simulink model "ATRIAS_vnmc"  (R2015a)
settings: Solver=ode45  StartTime=0.0  StopTime=60  FixedStep=1e-3  MinStep=1e-6  RelTol=1e-3  AbsTol=1e-4
values from neighbouring files (symbols this model uses):
  initial_boom_yaw = initial_boom_yaw + delta_yaw0    [run_model.m]
  max_floor_diff = cost_fun_opts.max_floor_diff    [opt_cmaes.m]    (also in run_model.m; set_all_params_simple.m = 0)
  noise_on_off = cost_fun_opts.noise_on_off    [opt_cmaes.m]    (also in run_model.m; set_all_params_simple.m = 0)
  noise_seed = cost_fun_opts.noise_seed    [opt_cmaes.m]    (also in run_model.m; set_all_params_simple.m = 1)
  noise_variance = cost_fun_opts.noise_variance    [opt_cmaes.m]    (also in run_model.m; set_all_params_simple.m = 0.000174532925199)
  SEA_swing_ctrl_on_off = cost_fun_opts.SEA_swing_ctrl_on_off    [opt_cmaes.m]    (also in run_model.m; set_all_params_simple.m = 0)
  sim_t = simout.twalk    [run_model.m]
  steady_dist = cost_fun_opts.steady_dist    [opt_cmaes.m]    (also in run_model.m; set_all_params_simple.m = 10)
  ts_anim = 0.0333    [run_model.m]
undefined symbols (not defined in the file or in its folder): A1_notch_f1, A2_notch_f1, A_lpf_dtau, A_lpf_velocity, B1_lpf_dtau, B1_lpf_velocity, B1_notch_f1, B2_lpf_dtau, B2_lpf_velocity, B2_notch_f1, b_hmotor, b_leg_spring, b_rotor, base_color_d, boom_color_d, boom_mount_to_center_diagonal, breakaway_friction, c, c_jointstop, com_height_offset, contactThr, coulomb_friction, CtrlPar_theta0, D12_S, D12_T, d_com, ddx_max, ddy_max, delta_phi_max, delta_phi_max_buffer, delta_phi_max_dropoff, delta_phi_min, des_forward_velocity, DS_width, dtau_des_max, dtheta0_vmc, dx0_vmc, dy_max, eref, fblink_color_d, fcut_acceleration, floor_color_d, floor_tile_width, floor_zero_height, FmaxBFSH, FmaxGLU, FmaxHAM, FmaxHFL, FmaxRF, FmaxVAS, FPCtrlPar, friction_linear_zone, g, gain_nodes_sea_torque, gamma_stance_thr, gamma_swing_thr, hip_height, HIP_MTR_MAX_CONT_TORQUE, HIP_MTR_MAX_TORQUE, hshaft_color_d ... (+236)
libraries: sm_lib x280, nesl_utility x174, simulink x114, simulink_extras x58, fl_lib x16, mblibv1 x2, dspswit3 x2
(part 23 of 23)

== matlab function ATRIAS_vnmc/control/Virtual Model Control/Swing Leg Behavior1/Avoid Hitting Mechanical Limits ==
  settings: updateMethod=DISCRETE  sampleTime=sample_time
  data: back_cmd output double; front_cmd output double; dback_cmd output double; dfront_cmd output double; ddback_cmd output double; ddfront_cmd output double; back_desired input; dback_desired input; ddback_desired input; front_desired input; dfront_desired input; ddfront_desired input; min_front_bar_angle parameter; max_front_bar_angle parameter; min_back_bar_angle parameter; max_back_bar_angle parameter
%% Avoid joint limits by ensuring we don't command velocities/accelerations that would push us into them when we are close to them.
function [back_cmd, front_cmd, dback_cmd, dfront_cmd, ddback_cmd, ddfront_cmd] ...
    = AvoidFourbarLimits(back_desired,dback_desired, ddback_desired, ...
          front_desired, dfront_desired, ddfront_desired, ...
          min_front_bar_angle, max_front_bar_angle, min_back_bar_angle, max_back_bar_angle)
    [back_cmd, front_cmd, dback_cmd, dfront_cmd, ddback_cmd, ddfront_cmd] = AvoidFourbarLimits(back_desired,dback_desired, ddback_desired, front_desired, dfront_desired, ddfront_desired, min_front_bar_angle, max_front_bar_angle, min_back_bar_angle, max_back_bar_angle);
end

== matlab function ATRIAS_vnmc/control/Virtual Model Control/Swing Leg Behavior1/Leg Angle Trajectory ==
  settings: updateMethod=DISCRETE  sampleTime=sample_time
  data: t input double; gamma_initial input double; gamma_final input double; t_trajectory input double; gamma output double; dgamma output double; ddgamma output double; max_gamma_velocity input; max_gamma_acceleration input
function [gamma, dgamma, ddgamma] = ...
    LegAngleTrajectory(t, gamma_initial, gamma_final, t_trajectory,...
                        max_gamma_velocity, max_gamma_acceleration)
                    
    t = max(0,t);    
    t_trajectory = max(0, t_trajectory);
    target_distance = gamma_final - gamma_initial;
    [t_ramp, t_hold] = ...
        trapezoidal_trajectory_max_time(t_trajectory, max_gamma_acceleration,...
        max_gamma_velocity, abs(target_distance));
    max_gamma_acceleration = max_gamma_acceleration*sign(target_distance);

    % generate trajectory
    if (t >= 0 && t <= t_ramp)
        gamma = gamma_initial + 0.5*max_gamma_acceleration*t^2;
        dgamma = max_gamma_acceleration*t;
        ddgamma = max_gamma_acceleration;
    elseif (t > t_ramp && t <= t_ramp+t_hold)
        gamma = gamma_initial + 0.5*max_gamma_acceleration*t_ramp^2 + (t-t_ramp)*max_gamma_acceleration*t_ramp;
        dgamma = max_gamma_acceleration*t_ramp;
        ddgamma = 0;
    elseif (t > t_ramp+t_hold && t <= t_hold + 2*t_ramp)
        gamma = gamma_initial + 0.5*max_gamma_acceleration*t_ramp^2 + t_hold*max_gamma_acceleration*t_ramp + ...
                max_gamma_acceleration*t_ramp*(t-t_ramp-t_hold) - 0.5*max_gamma_acceleration*(t-t_ramp-t_hold)^2;
        dgamma = max_gamma_acceleration*t_ramp - max_gamma_acceleration*(t-t_ramp-t_hold);
        ddgamma = -max_gamma_acceleration;
    else
        gamma = gamma_initial + max_gamma_acceleration*t_ramp^2 + max_gamma_acceleration*t_ramp*t_hold;
        dgamma = 0;
        ddgamma = 0;
    end
end

== matlab function ATRIAS_vnmc/control/Virtual Model Control/Swing Leg Behavior1/Leg Length Trajectory ==
  settings: updateMethod=DISCRETE  sampleTime=sample_time
  data: t input double size=1; l_leg_initial input double size=1; l_leg_final input double size=1; t_trajectory input double size=1; l_leg output double size=1; dl_leg output double size=1; ddl_leg output double size=1; max_leg_velocity input size=1; max_leg_acceleration input size=1
function [l_leg, dl_leg, ddl_leg] = ...
    LegAngleTrajectory(t, l_leg_initial, l_leg_final, t_trajectory,...
                        max_leg_velocity, max_leg_acceleration)
                    
    t = max(0,t);    
    t_trajectory = max(0, t_trajectory);
    target_distance = l_leg_final - l_leg_initial;
    [t_ramp, t_hold] = ...
        trapezoidal_trajectory_max_time(t_trajectory, max_leg_acceleration,...
        max_leg_velocity, abs(target_distance));
    max_leg_acceleration = max_leg_acceleration*sign(target_distance);

    % generate trajectory
    if (t >= 0 && t <= t_ramp)
        l_leg = l_leg_initial + 0.5*max_leg_acceleration*t^2;
        dl_leg = max_leg_acceleration*t;
        ddl_leg = max_leg_acceleration;
    elseif (t > t_ramp && t <= t_ramp+t_hold)
        l_leg = l_leg_initial + 0.5*max_leg_acceleration*t_ramp^2 + (t-t_ramp)*max_leg_acceleration*t_ramp;
        dl_leg = max_leg_acceleration*t_ramp;
        ddl_leg = 0;
    elseif (t > t_ramp+t_hold && t <= t_hold + 2*t_ramp)
        l_leg = l_leg_initial + 0.5*max_leg_acceleration*t_ramp^2 + t_hold*max_leg_acceleration*t_ramp + ...
                max_leg_acceleration*t_ramp*(t-t_ramp-t_hold) - 0.5*max_leg_acceleration*(t-t_ramp-t_hold)^2;
        dl_leg = max_leg_acceleration*t_ramp - max_leg_acceleration*(t-t_ramp-t_hold);
        ddl_leg = -max_leg_acceleration;
    else
        l_leg = l_leg_initial + max_leg_acceleration*t_ramp^2 + max_leg_acceleration*t_ramp*t_hold;
        dl_leg = 0;
        ddl_leg = 0;
    end
end

== matlab function ATRIAS_vnmc/control/Virtual Model Control/Swing Leg Behavior1/Virtual Leg to Four Bar ==
  settings: updateMethod=DISCRETE  sampleTime=sample_time
  data: l_leg input; dl_leg input; ddl_leg input; phi input; dphi input; ddphi input; back output; dback output; ddback output; front output; dfront output; ddfront output
function [back, dback, ddback, front, dfront, ddfront] = VirtualLegToFourBar(l_leg, dl_leg, ddl_leg, phi, dphi, ddphi)
    [back, dback, ddback, front, dfront, ddfront] = VirtualLegToFourBar(l_leg, dl_leg, ddl_leg, phi, dphi, ddphi);
end

== matlab function ATRIAS_vnmc/control/Virtual Model Control/Flight PD/Virtual Leg to Four Bar1 ==
  settings: updateMethod=DISCRETE  sampleTime=sample_time
  data: l_leg input; dl_leg input; ddl_leg input; phi input; dphi input; ddphi input; back output; dback output; ddback output; front output; dfront output; ddfront output
function [back, dback, ddback, front, dfront, ddfront] = VirtualLegToFourBar(l_leg, dl_leg, ddl_leg, phi, dphi, ddphi)
    [back, dback, ddback, front, dfront, ddfront] = VirtualLegToFourBar(l_leg, dl_leg, ddl_leg, phi, dphi, ddphi);
end

== matlab function ATRIAS_vnmc/control/Virtual Model Control/Flight PD/Avoid Hitting Mechanical Limits2 ==
  settings: updateMethod=DISCRETE  sampleTime=sample_time
  data: back_cmd output double; front_cmd output double; dback_cmd output double; dfront_cmd output double; ddback_cmd output double; ddfront_cmd output double; back_desired input; dback_desired input; ddback_desired input; front_desired input; dfront_desired input; ddfront_desired input; min_front_bar_angle parameter; max_front_bar_angle parameter; min_back_bar_angle parameter; max_back_bar_angle parameter
%% Avoid joint limits by ensuring we don't command velocities/accelerations that would push us into them when we are close to them.
function [back_cmd, front_cmd, dback_cmd, dfront_cmd, ddback_cmd, ddfront_cmd] ...
    = AvoidFourbarLimits(back_desired,dback_desired, ddback_desired, ...
          front_desired, dfront_desired, ddfront_desired, ...
          min_front_bar_angle, max_front_bar_angle, min_back_bar_angle, max_back_bar_angle)
    [back_cmd, front_cmd, dback_cmd, dfront_cmd, ddback_cmd, ddfront_cmd] = AvoidFourbarLimits(back_desired,dback_desired, ddback_desired, front_desired, dfront_desired, ddfront_desired, min_front_bar_angle, max_front_bar_angle, min_back_bar_angle, max_back_bar_angle);
end

== matlab function ATRIAS_vnmc/control/Virtual Model Control/Flight PD/Virtual Leg to Four Bar2 ==
  settings: updateMethod=DISCRETE  sampleTime=sample_time
  data: l_leg input; dl_leg input; ddl_leg input; phi input; dphi input; ddphi input; back output; dback output; ddback output; front output; dfront output; ddfront output
function [back, dback, ddback, front, dfront, ddfront] = VirtualLegToFourBar(l_leg, dl_leg, ddl_leg, phi, dphi, ddphi)
    [back, dback, ddback, front, dfront, ddfront] = VirtualLegToFourBar(l_leg, dl_leg, ddl_leg, phi, dphi, ddphi);
end

== matlab function ATRIAS_vnmc/control/Virtual Model Control/KKT_SS ==
  settings: updateMethod=DISCRETE  sampleTime=sample_time
  data: ddx_des input size=1; motor_trq output size=[2,1]; ddy_des input size=1; ddtheta_des input size=1; L input size=1; gamma input size=1; splay input size=1; theta input size=1; lambda1 input size=1; lambda2 input size=1; lambda3 input size=1; lambda4 input; mu_s input; grf_prev input size=[1,2]; leg_force_hip_torque output size=[2,1]; grf output size=[2,1]; cost_tie_break output size=1; err output size=[1,3]
function [motor_trq,leg_force_hip_torque,grf,cost_tie_break,err]  = ...
         vmc_SS(ddx_des,ddy_des,ddtheta_des,...
         L,gamma,splay,theta,lambda1,lambda2,lambda3,lambda4,mu_s,grf_prev)


m = 64;
I = 4;
d = 0.1;
l_seg = 0.5;
g = 9.81;
% mu_s = 0.25;

f1 = [(I*m*mu_s*(I*ddy_des*lambda2 + I*g*lambda2 + I*ddx_des*lambda1*mu_s - L*ddtheta_des*lambda3*m*sin(gamma) + d*ddtheta_des*lambda3*m*sin(theta) + L*ddtheta_des*lambda3*m*mu_s*cos(gamma) - d*ddtheta_des*lambda3*m*mu_s*cos(theta)))/(I^2*lambda2 + I^2*lambda1*mu_s^2 + L^2*lambda3*m^2*sin(gamma)^2 + d^2*lambda3*m^2*sin(theta)^2 + L^2*lambda3*m^2*mu_s^2*cos(gamma)^2 + d^2*lambda3*m^2*mu_s^2*cos(theta)^2 - 2*L*d*lambda3*m^2*sin(gamma)*sin(theta) - 2*L^2*lambda3*m^2*mu_s*cos(gamma)*sin(gamma) - 2*d^2*lambda3*m^2*mu_s*cos(theta)*sin(theta) + 2*L*d*lambda3*m^2*mu_s*cos(gamma)*sin(theta) + 2*L*d*lambda3*m^2*mu_s*cos(theta)*sin(gamma) - 2*L*d*lambda3*m^2*mu_s^2*cos(gamma)*cos(theta));
    -(I*m*mu_s*(I*ddy_des*lambda2 + I*g*lambda2 - I*ddx_des*lambda1*mu_s - L*ddtheta_des*lambda3*m*sin(gamma) + d*ddtheta_des*lambda3*m*sin(theta) - L*ddtheta_des*lambda3*m*mu_s*cos(gamma) + d*ddtheta_des*lambda3*m*mu_s*cos(theta)))/(I^2*lambda2 + I^2*lambda1*mu_s^2 + L^2*lambda3*m^2*sin(gamma)^2 + d^2*lambda3*m^2*sin(theta)^2 + L^2*lambda3*m^2*mu_s^2*cos(gamma)^2 + d^2*lambda3*m^2*mu_s^2*cos(theta)^2 - 2*L*d*lambda3*m^2*sin(gamma)*sin(theta) + 2*L^2*lambda3*m^2*mu_s*cos(gamma)*sin(gamma) + 2*d^2*lambda3*m^2*mu_s*cos(theta)*sin(theta) - 2*L*d*lambda3*m^2*mu_s*cos(gamma)*sin(theta) - 2*L*d*lambda3*m^2*mu_s*cos(theta)*sin(gamma) - 2*L*d*lambda3*m^2*mu_s^2*cos(gamma)*cos(theta));
    0;
    (I*m*(I*ddx_des*lambda1 + L*ddtheta_des*lambda3*m*cos(gamma) - d*ddtheta_des*lambda3*m*cos(theta)))/(I^2*lambda1 + L^2*lambda3*m^2*cos(gamma)^2 + d^2*lambda3*m^2*cos(theta)^2 - 2*L*d*lambda3*m^2*cos(gamma)*cos(theta));
    0;
    0;
    0;
    (I^2*ddx_des*lambda1*lambda2*m + L^2*ddx_des*lambda1*lambda3*m^3*sin(gamma)^2 + d^2*ddx_des*lambda1*lambda3*m^3*sin(theta)^2 + L^2*ddy_des*lambda2*lambda3*m^3*cos(gamma)*sin(gamma) + L^2*g*lambda2*lambda3*m^3*cos(gamma)*sin(gamma) + I*L*ddtheta_des*lambda2*lambda3*m^2*cos(gamma) + d^2*ddy_des*lambda2*lambda3*m^3*cos(theta)*sin(theta) - I*d*ddtheta_des*lambda2*lambda3*m^2*cos(theta) + d^2*g*lambda2*lambda3*m^3*cos(theta)*sin(theta) - L*d*ddy_des*lambda2*lambda3*m^3*cos(gamma)*sin(theta) - L*d*ddy_des*lambda2*lambda3*m^3*cos(theta)*sin(gamma) - L*d*g*lambda2*lambda3*m^3*cos(gamma)*sin(theta) - L*d*g*lambda2*lambda3*m^3*cos(theta)*sin(gamma) - 2*L*d*ddx_des*lambda1*lambda3*m^3*sin(gamma)*sin(theta))/(I^2*lambda1*lambda2 + d^2*lambda1*lambda3*m^2*sin(theta)^2 + L^2*lambda2*lambda3*m^2*cos(gamma)^2 + L^2*lambda1*lambda3*m^2*sin(gamma)^2 + d^2*lambda2*lambda3*m^2*cos(theta)^2 - 2*L*d*lambda2*lambda3*m^2*cos(gamma)*cos(theta) - 2*L*d*lambda1*lambda3*m^2*sin(gamma)*sin(theta))];

f2 = [(I*m*(I*ddy_des*lambda2 + I*g*lambda2 + I*ddx_des*lambda1*mu_s - L*ddtheta_des*lambda3*m*sin(gamma) + d*ddtheta_des*lambda3*m*sin(theta) + L*ddtheta_des*lambda3*m*mu_s*cos(gamma) - d*ddtheta_des*lambda3*m*mu_s*cos(theta)))/(I^2*lambda2 + I^2*lambda1*mu_s^2 + L^2*lambda3*m^2*sin(gamma)^2 + d^2*lambda3*m^2*sin(theta)^2 + L^2*lambda3*m^2*mu_s^2*cos(gamma)^2 + d^2*lambda3*m^2*mu_s^2*cos(theta)^2 - 2*L*d*lambda3*m^2*sin(gamma)*sin(theta) - 2*L^2*lambda3*m^2*mu_s*cos(gamma)*sin(gamma) - 2*d^2*lambda3*m^2*mu_s*cos(theta)*sin(theta) + 2*L*d*lambda3*m^2*mu_s*cos(gamma)*sin(theta) + 2*L*d*lambda3*m^2*mu_s*cos(theta)*sin(gamma) - 2*L*d*lambda3*m^2*mu_s^2*cos(gamma)*cos(theta));
    (I*m*(I*ddy_des*lambda2 + I*g*lambda2 - I*ddx_des*lambda1*mu_s - L*ddtheta_des*lambda3*m*sin(gamma) + d*ddtheta_des*lambda3*m*sin(theta) - L*ddtheta_des*lambda3*m*mu_s*cos(gamma) + d*ddtheta_des*lambda3*m*mu_s*cos(theta)))/(I^2*lambda2 + I^2*lambda1*mu_s^2 + L^2*lambda3*m^2*sin(gamma)^2 + d^2*lambda3*m^2*sin(theta)^2 + L^2*lambda3*m^2*mu_s^2*cos(gamma)^2 + d^2*lambda3*m^2*mu_s^2*cos(theta)^2 - 2*L*d*lambda3*m^2*sin(gamma)*sin(theta) + 2*L^2*lambda3*m^2*mu_s*cos(gamma)*sin(gamma) + 2*d^2*lambda3*m^2*mu_s*cos(theta)*sin(theta) - 2*L*d*lambda3*m^2*mu_s*cos(gamma)*sin(theta) - 2*L*d*lambda3*m^2*mu_s*cos(theta)*sin(gamma) - 2*L*d*lambda3*m^2*mu_s^2*cos(gamma)*cos(theta));
    0;
    0;
    0;
    0;
    0;
    (m*(I^2*ddy_des*lambda1*lambda2 + I^2*g*lambda1*lambda2 + L^2*ddy_des*lambda2*lambda3*m^2*cos(gamma)^2 + L^2*g*lambda2*lambda3*m^2*cos(gamma)^2 + d^2*ddy_des*lambda2*lambda3*m^2*cos(theta)^2 + d^2*g*lambda2*lambda3*m^2*cos(theta)^2 - I*L*ddtheta_des*lambda1*lambda3*m*sin(gamma) + I*d*ddtheta_des*lambda1*lambda3*m*sin(theta) + L^2*ddx_des*lambda1*lambda3*m^2*cos(gamma)*sin(gamma) + d^2*ddx_des*lambda1*lambda3*m^2*cos(theta)*sin(theta) - 2*L*d*ddy_des*lambda2*lambda3*m^2*cos(gamma)*cos(theta) - 2*L*d*g*lambda2*lambda3*m^2*cos(gamma)*cos(theta) - L*d*ddx_des*lambda1*lambda3*m^2*cos(gamma)*sin(theta) - L*d*ddx_des*lambda1*lambda3*m^2*cos(theta)*sin(gamma)))/(I^2*lambda1*lambda2 + d^2*lambda1*lambda3*m^2*sin(theta)^2 + L^2*lambda2*lambda3*m^2*cos(gamma)^2 + L^2*lambda1*lambda3*m^2*sin(gamma)^2 + d^2*lambda2*lambda3*m^2*cos(theta)^2 - 2*L*d*lambda2*lambda3*m^2*cos(gamma)*cos(theta) - 2*L*d*lambda1*lambda3*m^2*sin(gamma)*sin(theta))];

% numerical precision factor 
thr = 100*eps; % (without this, solution can give suboptimal/unexpected results)
c1 = mu_s*f2-f1 >= -thr;
c2 = mu_s*f2+f1 >= -thr;
c3 = f2 >= -thr;

constraints = c1 & c2 & c3;
satisfied = find(constraints);

ddx = 1/m*(f1);
ddy = 1/m*(f2-m*g);
ddtheta = 1/I*(f1*(-d*cos(theta)+L*cos(gamma))+f2*(d*sin(theta)-L*sin(gamma)));

% F1 = zeros(size(ddx));
% F2 = zeros(size(ddx));

F1 = lambda1*(ddx-ddx_des).^2+lambda2*(ddy-ddy_des).^2+lambda3*(ddtheta-ddtheta_des).^2;

% F1 = lambda1*(ddx-ddx_des).^2+lambda2*(ddy-ddy_des).^2+lambda3*(ddtheta-ddtheta_des).^2+...
%     lambda4*(abs(f1-grf_prev(1)) + abs(f2-grf_prev(2)));
% F2 = (f1-grf_prev(1)).^2 + (f2-grf_prev(2)).^2;
% F2 = (sign(f1)~= sign(grf_prev(1)))+(sign(f2)~= sign(grf_prev(2)));
F2 = abs(f1-grf_prev(1)) + abs(f2-grf_prev(2));

% F1 = F1(constraints);
% F2 = F2(constraints);



% if length(F1)>1
%     [F1_sorted,F1_sorted_idx] = sort(F1);
%     diff_F1_sorted = diff(F1_sorted);
%     same_cost_idx = find(diff_F1_sorted,1);
%     
%     if isempty(same_cost_idx)
%         same_cost_idx = length(F1_sorted_idx);
%     end
%     
%     [cost,min_idx] = min(F2(F1_sorted_idx(1:same_cost_idx(1))));
%     min_idx = F1_sorted_idx(min_idx);
% else
%     [cost,min_idx] = min(F1);
% end
[M,~] = min(F1(satisfied));
if ~isempty(M)
    I = satisfied(F1(satisfied)-M <= thr);
    [cost_tie_break, I2] = min(F2(I));
%     ddx_satisfied = ddx(constraints);
%     ddy_satisfied = ddy(constraints);
%     ddtheta_satisfied = ddtheta(constraints);
    
    e_ddx = ddx(I(I2)) - ddx_des;
    e_ddy = ddy(I(I2)) - ddy_des;
    e_ddtheta = ddtheta(I(I2)) - ddtheta_des;
%     e_ddx = ddx_satisfied(min_idx) - ddx_des;
%     e_ddy = ddy_satisfied(min_idx) - ddy_des;
%     e_ddtheta = ddtheta_satisfied(min_idx) - ddtheta_des;
    
    err = [e_ddx e_ddy e_ddtheta];
    
%     f1 = f1(constraints); f1 = f1(min_idx);
%     f2 = f2(constraints); f2 = f2(min_idx);
    f1 = f1(I(I2));
    f2 = f2(I(I2));

    grf = [f1; f2];
    
    J1 = [-sin(gamma) -cos(gamma);
        -L*cos(gamma) L*sin(gamma)];
    
    J2 = [-l_seg*sin(splay/2) 0.5;
        l_seg*sin(splay/2) 0.5];
    
    leg_force_hip_torque = J1*grf;
    motor_trq = J2*leg_force_hip_torque;
else
    grf = [0;0];
    err = [-ddx_des -ddy_des -ddtheta_des];
    leg_force_hip_torque = [0;0];
    motor_trq = [0;0];
end

end

== matlab function ATRIAS_vnmc/control/Virtual Model Control/Swing Leg Behavior2/Leg Angle Trajectory ==
  settings: updateMethod=DISCRETE  sampleTime=sample_time
  data: t input double; gamma_initial input double; gamma_final input double; t_trajectory input double; gamma output double; dgamma output double; ddgamma output double; max_gamma_velocity input; max_gamma_acceleration input
function [gamma, dgamma, ddgamma] = ...
    LegAngleTrajectory(t, gamma_initial, gamma_final, t_trajectory,...
                        max_gamma_velocity, max_gamma_acceleration)
                    
    t = max(0,t);    
    t_trajectory = max(0, t_trajectory);
    target_distance = gamma_final - gamma_initial;
    [t_ramp, t_hold] = ...
        trapezoidal_trajectory_max_time(t_trajectory, max_gamma_acceleration,...
        max_gamma_velocity, abs(target_distance));
    max_gamma_acceleration = max_gamma_acceleration*sign(target_distance);

    % generate trajectory
    if (t >= 0 && t <= t_ramp)
        gamma = gamma_initial + 0.5*max_gamma_acceleration*t^2;
        dgamma = max_gamma_acceleration*t;
        ddgamma = max_gamma_acceleration;
    elseif (t > t_ramp && t <= t_ramp+t_hold)
        gamma = gamma_initial + 0.5*max_gamma_acceleration*t_ramp^2 + (t-t_ramp)*max_gamma_acceleration*t_ramp;
        dgamma = max_gamma_acceleration*t_ramp;
        ddgamma = 0;
    elseif (t > t_ramp+t_hold && t <= t_hold + 2*t_ramp)
        gamma = gamma_initial + 0.5*max_gamma_acceleration*t_ramp^2 + t_hold*max_gamma_acceleration*t_ramp + ...
                max_gamma_acceleration*t_ramp*(t-t_ramp-t_hold) - 0.5*max_gamma_acceleration*(t-t_ramp-t_hold)^2;
        dgamma = max_gamma_acceleration*t_ramp - max_gamma_acceleration*(t-t_ramp-t_hold);
        ddgamma = -max_gamma_acceleration;
    else
        gamma = gamma_initial + max_gamma_acceleration*t_ramp^2 + max_gamma_acceleration*t_ramp*t_hold;
        dgamma = 0;
        ddgamma = 0;
    end
end

== matlab function ATRIAS_vnmc/control/Virtual Model Control/Double Support Geometry/DS geometry ==
  settings: updateMethod=DISCRETE  sampleTime=sample_time
  data: step_width input; L_min output; DS_width input; height input; L_max output; gamma_min output; gamma_max output
function [L_min,L_max,gamma_min,gamma_max] = convert_to_L_gamma(step_width,DS_width,height)

[L_min,L_max,gamma_min,gamma_max] = DS_geom(step_width,DS_width,height);

end

== matlab function ATRIAS_vnmc/control/Virtual Model Control/KKT_SS1 ==
  settings: updateMethod=DISCRETE  sampleTime=sample_time
  data: ddx_des input size=1; motor_trq output size=[2,1]; ddy_des input size=1; ddtheta_des input size=1; L input size=1; gamma input size=1; splay input size=1; theta input size=1; lambda1 input size=1; lambda2 input size=1; lambda3 input size=1; lambda4 input; mu_s input; grf_prev input size=[1,2]; leg_force_hip_torque output size=[2,1]; grf output size=[2,1]; cost_tie_break output size=1; err output size=[1,3]
function [motor_trq,leg_force_hip_torque,grf,cost_tie_break,err]  = ...
         vmc_SS(ddx_des,ddy_des,ddtheta_des,...
         L,gamma,splay,theta,lambda1,lambda2,lambda3,lambda4,mu_s,grf_prev)


m = 64;
I = 4;
d = 0.1;
l_seg = 0.5;
g = 9.81;
% mu_s = 0.25;

f1 = [(I*m*mu_s*(I*ddy_des*lambda2 + I*g*lambda2 + I*ddx_des*lambda1*mu_s - L*ddtheta_des*lambda3*m*sin(gamma) + d*ddtheta_des*lambda3*m*sin(theta) + L*ddtheta_des*lambda3*m*mu_s*cos(gamma) - d*ddtheta_des*lambda3*m*mu_s*cos(theta)))/(I^2*lambda2 + I^2*lambda1*mu_s^2 + L^2*lambda3*m^2*sin(gamma)^2 + d^2*lambda3*m^2*sin(theta)^2 + L^2*lambda3*m^2*mu_s^2*cos(gamma)^2 + d^2*lambda3*m^2*mu_s^2*cos(theta)^2 - 2*L*d*lambda3*m^2*sin(gamma)*sin(theta) - 2*L^2*lambda3*m^2*mu_s*cos(gamma)*sin(gamma) - 2*d^2*lambda3*m^2*mu_s*cos(theta)*sin(theta) + 2*L*d*lambda3*m^2*mu_s*cos(gamma)*sin(theta) + 2*L*d*lambda3*m^2*mu_s*cos(theta)*sin(gamma) - 2*L*d*lambda3*m^2*mu_s^2*cos(gamma)*cos(theta));
    -(I*m*mu_s*(I*ddy_des*lambda2 + I*g*lambda2 - I*ddx_des*lambda1*mu_s - L*ddtheta_des*lambda3*m*sin(gamma) + d*ddtheta_des*lambda3*m*sin(theta) - L*ddtheta_des*lambda3*m*mu_s*cos(gamma) + d*ddtheta_des*lambda3*m*mu_s*cos(theta)))/(I^2*lambda2 + I^2*lambda1*mu_s^2 + L^2*lambda3*m^2*sin(gamma)^2 + d^2*lambda3*m^2*sin(theta)^2 + L^2*lambda3*m^2*mu_s^2*cos(gamma)^2 + d^2*lambda3*m^2*mu_s^2*cos(theta)^2 - 2*L*d*lambda3*m^2*sin(gamma)*sin(theta) + 2*L^2*lambda3*m^2*mu_s*cos(gamma)*sin(gamma) + 2*d^2*lambda3*m^2*mu_s*cos(theta)*sin(theta) - 2*L*d*lambda3*m^2*mu_s*cos(gamma)*sin(theta) - 2*L*d*lambda3*m^2*mu_s*cos(theta)*sin(gamma) - 2*L*d*lambda3*m^2*mu_s^2*cos(gamma)*cos(theta));
    0;
    (I*m*(I*ddx_des*lambda1 + L*ddtheta_des*lambda3*m*cos(gamma) - d*ddtheta_des*lambda3*m*cos(theta)))/(I^2*lambda1 + L^2*lambda3*m^2*cos(gamma)^2 + d^2*lambda3*m^2*cos(theta)^2 - 2*L*d*lambda3*m^2*cos(gamma)*cos(theta));
    0;
    0;
    0;
    (I^2*ddx_des*lambda1*lambda2*m + L^2*ddx_des*lambda1*lambda3*m^3*sin(gamma)^2 + d^2*ddx_des*lambda1*lambda3*m^3*sin(theta)^2 + L^2*ddy_des*lambda2*lambda3*m^3*cos(gamma)*sin(gamma) + L^2*g*lambda2*lambda3*m^3*cos(gamma)*sin(gamma) + I*L*ddtheta_des*lambda2*lambda3*m^2*cos(gamma) + d^2*ddy_des*lambda2*lambda3*m^3*cos(theta)*sin(theta) - I*d*ddtheta_des*lambda2*lambda3*m^2*cos(theta) + d^2*g*lambda2*lambda3*m^3*cos(theta)*sin(theta) - L*d*ddy_des*lambda2*lambda3*m^3*cos(gamma)*sin(theta) - L*d*ddy_des*lambda2*lambda3*m^3*cos(theta)*sin(gamma) - L*d*g*lambda2*lambda3*m^3*cos(gamma)*sin(theta) - L*d*g*lambda2*lambda3*m^3*cos(theta)*sin(gamma) - 2*L*d*ddx_des*lambda1*lambda3*m^3*sin(gamma)*sin(theta))/(I^2*lambda1*lambda2 + d^2*lambda1*lambda3*m^2*sin(theta)^2 + L^2*lambda2*lambda3*m^2*cos(gamma)^2 + L^2*lambda1*lambda3*m^2*sin(gamma)^2 + d^2*lambda2*lambda3*m^2*cos(theta)^2 - 2*L*d*lambda2*lambda3*m^2*cos(gamma)*cos(theta) - 2*L*d*lambda1*lambda3*m^2*sin(gamma)*sin(theta))];

f2 = [(I*m*(I*ddy_des*lambda2 + I*g*lambda2 + I*ddx_des*lambda1*mu_s - L*ddtheta_des*lambda3*m*sin(gamma) + d*ddtheta_des*lambda3*m*sin(theta) + L*ddtheta_des*lambda3*m*mu_s*cos(gamma) - d*ddtheta_des*lambda3*m*mu_s*cos(theta)))/(I^2*lambda2 + I^2*lambda1*mu_s^2 + L^2*lambda3*m^2*sin(gamma)^2 + d^2*lambda3*m^2*sin(theta)^2 + L^2*lambda3*m^2*mu_s^2*cos(gamma)^2 + d^2*lambda3*m^2*mu_s^2*cos(theta)^2 - 2*L*d*lambda3*m^2*sin(gamma)*sin(theta) - 2*L^2*lambda3*m^2*mu_s*cos(gamma)*sin(gamma) - 2*d^2*lambda3*m^2*mu_s*cos(theta)*sin(theta) + 2*L*d*lambda3*m^2*mu_s*cos(gamma)*sin(theta) + 2*L*d*lambda3*m^2*mu_s*cos(theta)*sin(gamma) - 2*L*d*lambda3*m^2*mu_s^2*cos(gamma)*cos(theta));
    (I*m*(I*ddy_des*lambda2 + I*g*lambda2 - I*ddx_des*lambda1*mu_s - L*ddtheta_des*lambda3*m*sin(gamma) + d*ddtheta_des*lambda3*m*sin(theta) - L*ddtheta_des*lambda3*m*mu_s*cos(gamma) + d*ddtheta_des*lambda3*m*mu_s*cos(theta)))/(I^2*lambda2 + I^2*lambda1*mu_s^2 + L^2*lambda3*m^2*sin(gamma)^2 + d^2*lambda3*m^2*sin(theta)^2 + L^2*lambda3*m^2*mu_s^2*cos(gamma)^2 + d^2*lambda3*m^2*mu_s^2*cos(theta)^2 - 2*L*d*lambda3*m^2*sin(gamma)*sin(theta) + 2*L^2*lambda3*m^2*mu_s*cos(gamma)*sin(gamma) + 2*d^2*lambda3*m^2*mu_s*cos(theta)*sin(theta) - 2*L*d*lambda3*m^2*mu_s*cos(gamma)*sin(theta) - 2*L*d*lambda3*m^2*mu_s*cos(theta)*sin(gamma) - 2*L*d*lambda3*m^2*mu_s^2*cos(gamma)*cos(theta));
    0;
    0;
    0;
    0;
    0;
    (m*(I^2*ddy_des*lambda1*lambda2 + I^2*g*lambda1*lambda2 + L^2*ddy_des*lambda2*lambda3*m^2*cos(gamma)^2 + L^2*g*lambda2*lambda3*m^2*cos(gamma)^2 + d^2*ddy_des*lambda2*lambda3*m^2*cos(theta)^2 + d^2*g*lambda2*lambda3*m^2*cos(theta)^2 - I*L*ddtheta_des*lambda1*lambda3*m*sin(gamma) + I*d*ddtheta_des*lambda1*lambda3*m*sin(theta) + L^2*ddx_des*lambda1*lambda3*m^2*cos(gamma)*sin(gamma) + d^2*ddx_des*lambda1*lambda3*m^2*cos(theta)*sin(theta) - 2*L*d*ddy_des*lambda2*lambda3*m^2*cos(gamma)*cos(theta) - 2*L*d*g*lambda2*lambda3*m^2*cos(gamma)*cos(theta) - L*d*ddx_des*lambda1*lambda3*m^2*cos(gamma)*sin(theta) - L*d*ddx_des*lambda1*lambda3*m^2*cos(theta)*sin(gamma)))/(I^2*lambda1*lambda2 + d^2*lambda1*lambda3*m^2*sin(theta)^2 + L^2*lambda2*lambda3*m^2*cos(gamma)^2 + L^2*lambda1*lambda3*m^2*sin(gamma)^2 + d^2*lambda2*lambda3*m^2*cos(theta)^2 - 2*L*d*lambda2*lambda3*m^2*cos(gamma)*cos(theta) - 2*L*d*lambda1*lambda3*m^2*sin(gamma)*sin(theta))];

% numerical precision factor 
thr = 100*eps; % (without this, solution can give suboptimal/unexpected results)
c1 = mu_s*f2-f1 >= -thr;
c2 = mu_s*f2+f1 >= -thr;
c3 = f2 >= -thr;

constraints = c1 & c2 & c3;
satisfied = find(constraints);

ddx = 1/m*(f1);
ddy = 1/m*(f2-m*g);
ddtheta = 1/I*(f1*(-d*cos(theta)+L*cos(gamma))+f2*(d*sin(theta)-L*sin(gamma)));

% F1 = zeros(size(ddx));
% F2 = zeros(size(ddx));

F1 = lambda1*(ddx-ddx_des).^2+lambda2*(ddy-ddy_des).^2+lambda3*(ddtheta-ddtheta_des).^2;

% F1 = lambda1*(ddx-ddx_des).^2+lambda2*(ddy-ddy_des).^2+lambda3*(ddtheta-ddtheta_des).^2+...
%     lambda4*(abs(f1-grf_prev(1)) + abs(f2-grf_prev(2)));
% F2 = (f1-grf_prev(1)).^2 + (f2-grf_prev(2)).^2;
% F2 = (sign(f1)~= sign(grf_prev(1)))+(sign(f2)~= sign(grf_prev(2)));
F2 = abs(f1-grf_prev(1)) + abs(f2-grf_prev(2));

% F1 = F1(constraints);
% F2 = F2(constraints);



% if length(F1)>1
%     [F1_sorted,F1_sorted_idx] = sort(F1);
%     diff_F1_sorted = diff(F1_sorted);
%     same_cost_idx = find(diff_F1_sorted,1);
%     
%     if isempty(same_cost_idx)
%         same_cost_idx = length(F1_sorted_idx);
%     end
%     
%     [cost,min_idx] = min(F2(F1_sorted_idx(1:same_cost_idx(1))));
%     min_idx = F1_sorted_idx(min_idx);
% else
%     [cost,min_idx] = min(F1);
% end
[M,~] = min(F1(satisfied));
if ~isempty(M)
    I = satisfied(F1(satisfied)-M <= thr);
    [cost_tie_break, I2] = min(F2(I));
%     ddx_satisfied = ddx(constraints);
%     ddy_satisfied = ddy(constraints);
%     ddtheta_satisfied = ddtheta(constraints);
    
    e_ddx = ddx(I(I2)) - ddx_des;
    e_ddy = ddy(I(I2)) - ddy_des;
    e_ddtheta = ddtheta(I(I2)) - ddtheta_des;
%     e_ddx = ddx_satisfied(min_idx) - ddx_des;
%     e_ddy = ddy_satisfied(min_idx) - ddy_des;
%     e_ddtheta = ddtheta_satisfied(min_idx) - ddtheta_des;
    
    err = [e_ddx e_ddy e_ddtheta];
    
%     f1 = f1(constraints); f1 = f1(min_idx);
%     f2 = f2(constraints); f2 = f2(min_idx);
    f1 = f1(I(I2));
    f2 = f2(I(I2));

    grf = [f1; f2];
    
    J1 = [-sin(gamma) -cos(gamma);
        -L*cos(gamma) L*sin(gamma)];
    
    J2 = [-l_seg*sin(splay/2) 0.5;
        l_seg*sin(splay/2) 0.5];
    
    leg_force_hip_torque = J1*grf;
    motor_trq = J2*leg_force_hip_torque;
else
    grf = [0;0];
    err = [-ddx_des -ddy_des -ddtheta_des];
    leg_force_hip_torque = [0;0];
    motor_trq = [0;0];
end

end

== matlab function ATRIAS_vnmc/control/Virtual Model Control/Swing Leg Behavior2/Avoid Hitting Mechanical Limits ==
  settings: updateMethod=DISCRETE  sampleTime=sample_time
  data: back_cmd output double; front_cmd output double; dback_cmd output double; dfront_cmd output double; ddback_cmd output double; ddfront_cmd output double; back_desired input; dback_desired input; ddback_desired input; front_desired input; dfront_desired input; ddfront_desired input; min_front_bar_angle parameter; max_front_bar_angle parameter; min_back_bar_angle parameter; max_back_bar_angle parameter
%% Avoid joint limits by ensuring we don't command velocities/accelerations that would push us into them when we are close to them.
function [back_cmd, front_cmd, dback_cmd, dfront_cmd, ddback_cmd, ddfront_cmd] ...
    = AvoidFourbarLimits(back_desired,dback_desired, ddback_desired, ...
          front_desired, dfront_desired, ddfront_desired, ...
          min_front_bar_angle, max_front_bar_angle, min_back_bar_angle, max_back_bar_angle)
    [back_cmd, front_cmd, dback_cmd, dfront_cmd, ddback_cmd, ddfront_cmd] = AvoidFourbarLimits(back_desired,dback_desired, ddback_desired, front_desired, dfront_desired, ddfront_desired, min_front_bar_angle, max_front_bar_angle, min_back_bar_angle, max_back_bar_angle);
end

== matlab function ATRIAS_vnmc/control/Virtual Model Control/COM PD Law/Min-time y_com trajectory ==
  settings: updateMethod=DISCRETE  sampleTime=sample_time
  data: t input double size=1; l_leg_initial input double size=1; l_leg_final input double size=1; t_trajectory input double size=1; l_leg output double size=1; dl_leg output double size=1; ddl_leg output double size=1; max_leg_velocity input size=1; max_leg_acceleration input size=1
function [l_leg, dl_leg, ddl_leg] = ...
    y_com_trajectory(t, l_leg_initial, l_leg_final, t_trajectory,...
                        max_leg_velocity, max_leg_acceleration)
                    
    t = max(0,t);    
    t_trajectory = max(0, t_trajectory);
    target_distance = l_leg_final - l_leg_initial;
    [t_ramp, t_hold] = ...
        trapezoidal_trajectory_max_time(t_trajectory, max_leg_acceleration,...
        max_leg_velocity, abs(target_distance));
    max_leg_acceleration = max_leg_acceleration*sign(target_distance);

    % generate trajectory
    if (t >= 0 && t <= t_ramp)
        l_leg = l_leg_initial + 0.5*max_leg_acceleration*t^2;
        dl_leg = max_leg_acceleration*t;
        ddl_leg = max_leg_acceleration;
    elseif (t > t_ramp && t <= t_ramp+t_hold)
        l_leg = l_leg_initial + 0.5*max_leg_acceleration*t_ramp^2 + (t-t_ramp)*max_leg_acceleration*t_ramp;
        dl_leg = max_leg_acceleration*t_ramp;
        ddl_leg = 0;
    elseif (t > t_ramp+t_hold && t <= t_hold + 2*t_ramp)
        l_leg = l_leg_initial + 0.5*max_leg_acceleration*t_ramp^2 + t_hold*max_leg_acceleration*t_ramp + ...
                max_leg_acceleration*t_ramp*(t-t_ramp-t_hold) - 0.5*max_leg_acceleration*(t-t_ramp-t_hold)^2;
        dl_leg = max_leg_acceleration*t_ramp - max_leg_acceleration*(t-t_ramp-t_hold);
        ddl_leg = -max_leg_acceleration;
    else
        l_leg = l_leg_initial + max_leg_acceleration*t_ramp^2 + max_leg_acceleration*t_ramp*t_hold;
        dl_leg = 0;
        ddl_leg = 0;
    end
end

== matlab function ATRIAS_vnmc/control/Virtual Model Control/Swing Leg Behavior2/Leg Length Trajectory ==
  settings: updateMethod=DISCRETE  sampleTime=sample_time
  data: t input double size=1; l_leg_initial input double size=1; l_leg_final input double size=1; t_trajectory input double size=1; l_leg output double size=1; dl_leg output double size=1; ddl_leg output double size=1; max_leg_velocity input size=1; max_leg_acceleration input size=1
function [l_leg, dl_leg, ddl_leg] = ...
    LegAngleTrajectory(t, l_leg_initial, l_leg_final, t_trajectory,...
                        max_leg_velocity, max_leg_acceleration)
                    
    t = max(0,t);    
    t_trajectory = max(0, t_trajectory);
    target_distance = l_leg_final - l_leg_initial;
    [t_ramp, t_hold] = ...
        trapezoidal_trajectory_max_time(t_trajectory, max_leg_acceleration,...
        max_leg_velocity, abs(target_distance));
    max_leg_acceleration = max_leg_acceleration*sign(target_distance);

    % generate trajectory
    if (t >= 0 && t <= t_ramp)
        l_leg = l_leg_initial + 0.5*max_leg_acceleration*t^2;
        dl_leg = max_leg_acceleration*t;
        ddl_leg = max_leg_acceleration;
    elseif (t > t_ramp && t <= t_ramp+t_hold)
        l_leg = l_leg_initial + 0.5*max_leg_acceleration*t_ramp^2 + (t-t_ramp)*max_leg_acceleration*t_ramp;
        dl_leg = max_leg_acceleration*t_ramp;
        ddl_leg = 0;
    elseif (t > t_ramp+t_hold && t <= t_hold + 2*t_ramp)
        l_leg = l_leg_initial + 0.5*max_leg_acceleration*t_ramp^2 + t_hold*max_leg_acceleration*t_ramp + ...
                max_leg_acceleration*t_ramp*(t-t_ramp-t_hold) - 0.5*max_leg_acceleration*(t-t_ramp-t_hold)^2;
        dl_leg = max_leg_acceleration*t_ramp - max_leg_acceleration*(t-t_ramp-t_hold);
        ddl_leg = -max_leg_acceleration;
    else
        l_leg = l_leg_initial + max_leg_acceleration*t_ramp^2 + max_leg_acceleration*t_ramp*t_hold;
        dl_leg = 0;
        ddl_leg = 0;
    end
end

== matlab function ATRIAS_vnmc/control/Virtual Model Control/Swing Leg Behavior2/Virtual Leg to Four Bar ==
  settings: updateMethod=DISCRETE  sampleTime=sample_time
  data: l_leg input; dl_leg input; ddl_leg input; phi input; dphi input; ddphi input; back output; dback output; ddback output; front output; dfront output; ddfront output
function [back, dback, ddback, front, dfront, ddfront] = VirtualLegToFourBar(l_leg, dl_leg, ddl_leg, phi, dphi, ddphi)
    [back, dback, ddback, front, dfront, ddfront] = VirtualLegToFourBar(l_leg, dl_leg, ddl_leg, phi, dphi, ddphi);
end

== matlab function ATRIAS_vnmc/control/Virtual Model Control/Swing Leg Behavior3/Avoid Hitting Mechanical Limits ==
  settings: updateMethod=DISCRETE  sampleTime=sample_time
  data: back_cmd output double; front_cmd output double; dback_cmd output double; dfront_cmd output double; ddback_cmd output double; ddfront_cmd output double; back_desired input; dback_desired input; ddback_desired input; front_desired input; dfront_desired input; ddfront_desired input; min_front_bar_angle parameter; max_front_bar_angle parameter; min_back_bar_angle parameter; max_back_bar_angle parameter
%% Avoid joint limits by ensuring we don't command velocities/accelerations that would push us into them when we are close to them.
function [back_cmd, front_cmd, dback_cmd, dfront_cmd, ddback_cmd, ddfront_cmd] ...
    = AvoidFourbarLimits(back_desired,dback_desired, ddback_desired, ...
          front_desired, dfront_desired, ddfront_desired, ...
          min_front_bar_angle, max_front_bar_angle, min_back_bar_angle, max_back_bar_angle)
    [back_cmd, front_cmd, dback_cmd, dfront_cmd, ddback_cmd, ddfront_cmd] = AvoidFourbarLimits(back_desired,dback_desired, ddback_desired, front_desired, dfront_desired, ddfront_desired, min_front_bar_angle, max_front_bar_angle, min_back_bar_angle, max_back_bar_angle);
end

== matlab function ATRIAS_vnmc/control/Virtual Model Control/Swing Leg Behavior3/Leg Angle Trajectory ==
  settings: updateMethod=DISCRETE  sampleTime=sample_time
  data: t input double; gamma_initial input double; gamma_final input double; t_trajectory input double; gamma output double; dgamma output double; ddgamma output double; max_gamma_velocity input; max_gamma_acceleration input
function [gamma, dgamma, ddgamma] = ...
    LegAngleTrajectory(t, gamma_initial, gamma_final, t_trajectory,...
                        max_gamma_velocity, max_gamma_acceleration)
                    
    t = max(0,t);    
    t_trajectory = max(0, t_trajectory);
    target_distance = gamma_final - gamma_initial;
    [t_ramp, t_hold] = ...
        trapezoidal_trajectory_max_time(t_trajectory, max_gamma_acceleration,...
        max_gamma_velocity, abs(target_distance));
    max_gamma_acceleration = max_gamma_acceleration*sign(target_distance);

    % generate trajectory
    if (t >= 0 && t <= t_ramp)
        gamma = gamma_initial + 0.5*max_gamma_acceleration*t^2;
        dgamma = max_gamma_acceleration*t;
        ddgamma = max_gamma_acceleration;
    elseif (t > t_ramp && t <= t_ramp+t_hold)
        gamma = gamma_initial + 0.5*max_gamma_acceleration*t_ramp^2 + (t-t_ramp)*max_gamma_acceleration*t_ramp;
        dgamma = max_gamma_acceleration*t_ramp;
        ddgamma = 0;
    elseif (t > t_ramp+t_hold && t <= t_hold + 2*t_ramp)
        gamma = gamma_initial + 0.5*max_gamma_acceleration*t_ramp^2 + t_hold*max_gamma_acceleration*t_ramp + ...
                max_gamma_acceleration*t_ramp*(t-t_ramp-t_hold) - 0.5*max_gamma_acceleration*(t-t_ramp-t_hold)^2;
        dgamma = max_gamma_acceleration*t_ramp - max_gamma_acceleration*(t-t_ramp-t_hold);
        ddgamma = -max_gamma_acceleration;
    else
        gamma = gamma_initial + max_gamma_acceleration*t_ramp^2 + max_gamma_acceleration*t_ramp*t_hold;
        dgamma = 0;
        ddgamma = 0;
    end
end

== matlab function ATRIAS_vnmc/control/Virtual Model Control/Swing Leg Behavior3/Leg Length Trajectory ==
  settings: updateMethod=DISCRETE  sampleTime=sample_time
  data: t input double size=1; l_leg_initial input double size=1; l_leg_final input double size=1; t_trajectory input double size=1; l_leg output double size=1; dl_leg output double size=1; ddl_leg output double size=1; max_leg_velocity input size=1; max_leg_acceleration input size=1
function [l_leg, dl_leg, ddl_leg] = ...
    LegAngleTrajectory(t, l_leg_initial, l_leg_final, t_trajectory,...
                        max_leg_velocity, max_leg_acceleration)
                    
    t = max(0,t);    
    t_trajectory = max(0, t_trajectory);
    target_distance = l_leg_final - l_leg_initial;
    [t_ramp, t_hold] = ...
        trapezoidal_trajectory_max_time(t_trajectory, max_leg_acceleration,...
        max_leg_velocity, abs(target_distance));
    max_leg_acceleration = max_leg_acceleration*sign(target_distance);

    % generate trajectory
    if (t >= 0 && t <= t_ramp)
        l_leg = l_leg_initial + 0.5*max_leg_acceleration*t^2;
        dl_leg = max_leg_acceleration*t;
        ddl_leg = max_leg_acceleration;
    elseif (t > t_ramp && t <= t_ramp+t_hold)
        l_leg = l_leg_initial + 0.5*max_leg_acceleration*t_ramp^2 + (t-t_ramp)*max_leg_acceleration*t_ramp;
        dl_leg = max_leg_acceleration*t_ramp;
        ddl_leg = 0;
    elseif (t > t_ramp+t_hold && t <= t_hold + 2*t_ramp)
        l_leg = l_leg_initial + 0.5*max_leg_acceleration*t_ramp^2 + t_hold*max_leg_acceleration*t_ramp + ...
                max_leg_acceleration*t_ramp*(t-t_ramp-t_hold) - 0.5*max_leg_acceleration*(t-t_ramp-t_hold)^2;
        dl_leg = max_leg_acceleration*t_ramp - max_leg_acceleration*(t-t_ramp-t_hold);
        ddl_leg = -max_leg_acceleration;
    else
        l_leg = l_leg_initial + max_leg_acceleration*t_ramp^2 + max_leg_acceleration*t_ramp*t_hold;
        dl_leg = 0;
        ddl_leg = 0;
    end
end

== matlab function ATRIAS_vnmc/control/Virtual Model Control/Swing Leg Behavior3/Virtual Leg to Four Bar ==
  settings: updateMethod=DISCRETE  sampleTime=sample_time
  data: l_leg input; dl_leg input; ddl_leg input; phi input; dphi input; ddphi input; back output; dback output; ddback output; front output; dfront output; ddfront output
function [back, dback, ddback, front, dfront, ddfront] = VirtualLegToFourBar(l_leg, dl_leg, ddl_leg, phi, dphi, ddphi)
    [back, dback, ddback, front, dfront, ddfront] = VirtualLegToFourBar(l_leg, dl_leg, ddl_leg, phi, dphi, ddphi);
end

== matlab function ATRIAS_vnmc/control/Lateral Motor Control/Lateral Control1 ==
  data: winch_unloaded input; tau_r output size=1; qLateralR input; dqLateralR input; qLateralL input; dqLateralL input; F_leg_R input; F_leg_L input; lateral_transition_force parameter; lateral_target_angle_right parameter; m_leg_motor parameter; m_leg parameter; m_total parameter; g parameter; lateral_offset parameter; tau_l output size=1; kp_lateral parameter; kd_lateral parameter; minimum_lateral_angle parameter; maximum_lateral_angle parameter; HIP_MTR_MAX_CONT_TORQUE parameter
function [tau_r, tau_l] = LateralBoomControl(winch_unloaded,...
    qLateralR, dqLateralR, qLateralL, dqLateralL, F_leg_R, F_leg_L,...
    lateral_transition_force, lateral_target_angle_right,...
    m_leg_motor, m_leg, m_total, g, lateral_offset,...
    kp_lateral, kd_lateral, minimum_lateral_angle, maximum_lateral_angle, HIP_MTR_MAX_CONT_TORQUE)
    
    % Only add gravity compensation to PD when suspended from winch (approximately static)
    gravity_compensation = 0;
    if ~winch_unloaded, gravity_compensation = (m_leg_motor+m_leg)*g*lateral_offset; end
    
    % Inertia for feedforward accelerations
    motor_inertia = (m_leg_motor+m_leg)*lateral_offset^2;
    
    % Right Leg
    right_target = [lateral_target_angle_right, 0, 0];
    desired = [saturate(right_target(1),minimum_lateral_angle,maximum_lateral_angle), right_target(2)];
    measured = [qLateralR, dqLateralR];
    tau_r = [kp_lateral, kd_lateral] * (desired-measured)' + gravity_compensation + motor_inertia*right_target(3);
    tau_r = max(min(HIP_MTR_MAX_CONT_TORQUE, tau_r),-HIP_MTR_MAX_CONT_TORQUE);
    
    if (F_leg_R >= lateral_transition_force)
        if winch_unloaded
            tau_r = -F_leg_R*lateral_offset*(m_total-(m_leg_motor+m_leg))/m_total + ...
                    F_leg_L*lateral_offset*((m_leg_motor+m_leg)/m_total);
        else
            tau_r = -lateral_offset*(F_leg_R-(m_leg_motor+m_leg)*g);
        end
    end
    
    % Left Leg
    left_target = [lateral_target_angle_right, 0, 0];
    desired = [saturate(left_target(1),minimum_lateral_angle,maximum_lateral_angle), left_target(2)];
    measured = [qLateralL, dqLateralL];
    tau_l = [kp_lateral, kd_lateral] * (desired-measured)' + gravity_compensation + motor_inertia*left_target(3);
    tau_l = max(min(HIP_MTR_MAX_CONT_TORQUE, tau_l),-HIP_MTR_MAX_CONT_TORQUE);
    
    if (F_leg_L >= lateral_transition_force)
        if winch_unloaded
            tau_l = -F_leg_L*lateral_offset*(m_total-(m_leg_motor+m_leg))/m_total + ...
                    F_leg_R*lateral_offset*((m_leg_motor+m_leg)/m_total);
        else
            tau_l = -lateral_offset*(F_leg_L-(m_leg_motor+m_leg)*g);
        end
    end
end

function [desired_saturated] = saturate(desired, minimum_lateral_angle, maximum_lateral_angle)
    desired_saturated = desired;
    if desired(1) < minimum_lateral_angle
        desired_saturated = [minimum_lateral_angle, 0];
    elseif desired(1) > maximum_lateral_angle
        desired_saturated = [maximum_lateral_angle, 0];    
    end
end
